simulink model "diff_controller"  (R2024b)
settings: Solver=FixedStepAuto  StartTime=0.0  StopTime=inf  FixedStep=0.001  RelTol=1e-3  EnableMultiTasking=on
InitFcn:
  | Ts = 0.005;
  | diameter = 165; %mm
  | width = 441; %mm
libraries: arduinolib x19, simulink x10, svdutilitieslib x5, simulink_extras x3, arduinosensorlib x2, robotmobilelib x1
(part 1 of 2)
settings Model: ExtModeTrigDuration=2  Creator=System-10  LastModifiedBy=01149
settings SolverCC: AutoInsertRateTranBlk=on
settings OptimizationCC: EnhancedBackFolding=on  PassReuseOutputArgsAs=Individual arguments  ZeroExternalMemoryAtStartup=off  ZeroInternalMemoryAtStartup=off  MaxStackSize=64  OptimizeBlockOrder=speed  DifferentSizesBufferReuse=on  OptimizationCustomize=off  EfficientTunableParamExpr=on
settings DebuggingCC: ParameterTunabilityLossMsg=error
settings HardwareCC: ProdBitPerInt=16  ProdBitPerPointer=16  ProdBitPerSizeT=16  ProdBitPerPtrDiffT=16  ProdLargestAtomicFloat=None  ProdWordSize=8  ProdHWDeviceType=Atmel->AVR
settings SFSimCC: MATLABDynamicMemAlloc=off
settings RTWCC: Description=Embedded Coder  SystemTargetFile=ert.tlc  HardwareBoard=Arduino Mega 2560  TemplateMakefile=ert_default_tmf  GenerateReport=on  Toolchain=Arduino AVR  BuildConfiguration=Faster Runs  GPUComputeCapability=3.5
settings CodeAppCC: ForceParamTrailComments=on  IgnoreCustomStorageClasses=off  OperatorAnnotations=on  SimulinkDataObjDesc=on  SFDataObjDesc=on  InsertBlockDesc=on
settings ERTTargetCC: SupportContinuousTime=on  SupportVariableSizeSignals=on  ExtModeTransport=3  ExtModeStaticAlloc=on  ExtModeAutomaticAllocSize=off  ExtModeStaticAllocSize=2048  ExtModeMexFile=ext_xcp  ExtModeIntrfLevel=Level2 - Open  InlinedParameterPlacement=Hierarchical  DynamicArrayContainerType=coder::array

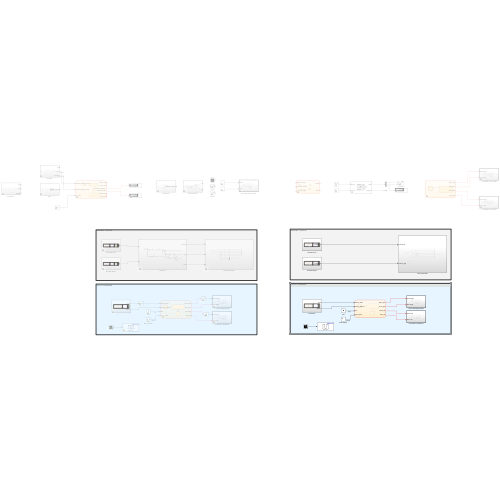
[thumbnail: Simulink's stored preview of the top-level diagram]
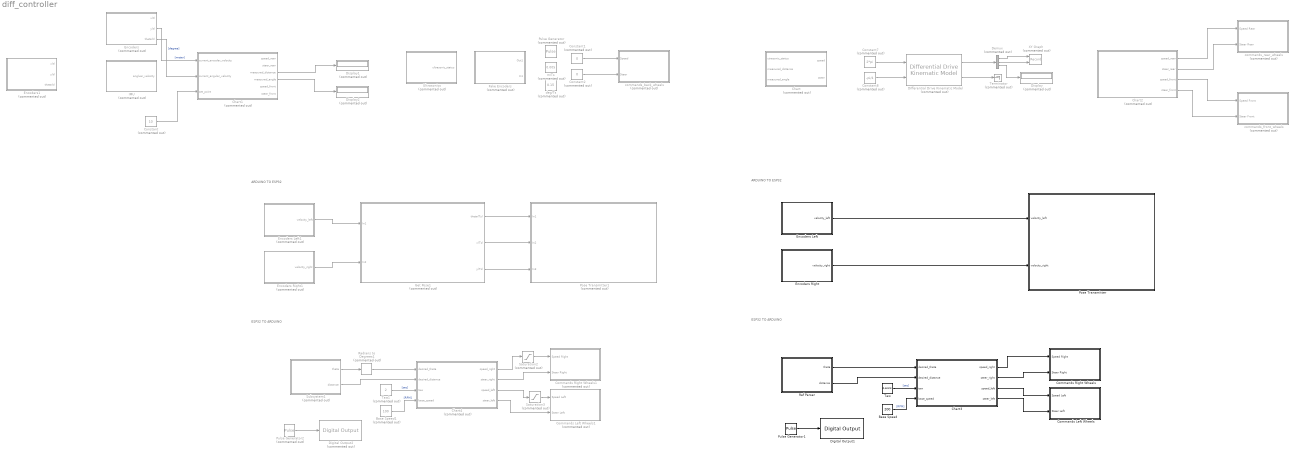
== system diff_controller ==
  note: ARDUINO TO ESP32
  note: ESP32 TO ARDUINO
  note: ESP32 TO ARDUINO
  note: ARDUINO TO ESP32
  Base Speed : Constant  Value=200  SampleTime=Ts
  Base Speed1 : Constant  Commented=on  Value=100  SampleTime=Ts
  Chart : Stateflow chart  Commented=on  TreatAsAtomicUnit=on
  Chart1 : Stateflow chart  Commented=on  TreatAsAtomicUnit=on
      settings: PortSchema="{\"entries\":[{\"content\":{\"sides\":[{\"content\":{\"connectorIds\":[\"In1\",\"In2\",\"In3\"]},\"type\":\"ConnectorPlacement.EquallySpacedRectSide\",\"uuid\":\"a18cf0c3-3c77-458c-bb3e-450a9e5c4723\"},{\"content\":{\"connectorIds\":[\"Out1\",\"Out2\",\"Out3\",\"Out6\",\"Out4\",\"Out5\"],\"side\":\"RIGHT\"},\"type\":\"ConnectorPlacement.EquallySpacedRectSide\",\"uuid\":\"c8115a23-9c0e-4673-86fd-819843dfe009\"},{\"content\":{\"side\":\"TOP\"},\"type\":\"ConnectorPlacement.EquallySpacedRectSide\",\"uuid\":\"db8a9c60-5937-48dc-b510-5b8795ac680a\"}]},\"type\":\"ConnectorPlacement.EquallySpacedConnector\",\"uuid\":\"4f3d77b9-4394-4090-867a-c6b2685c3613\"}],\"packageUris\":[\"http://schema.mathworks.com/mf0/Connector/R2020b\"],\"version\":\"1.0\"}"
  Chart2 : Stateflow chart  Commented=on  TreatAsAtomicUnit=on
  Chart3 : Stateflow chart  TreatAsAtomicUnit=on
  Chart4 : Stateflow chart  Commented=on  TreatAsAtomicUnit=on
  Commands Left Wheels : Subsystem  TreatAsAtomicUnit=on  SystemSampleTime=Ts
  Commands Left Wheels1 : Subsystem  Commented=on  TreatAsAtomicUnit=on  SystemSampleTime=0.1
  Commands Right Wheels : Subsystem  TreatAsAtomicUnit=on  SystemSampleTime=Ts
  Commands Right Wheels1 : Subsystem  Commented=on  TreatAsAtomicUnit=on  SystemSampleTime=0.1
  Constant : Constant  Commented=on  Value=10  SampleTime=Ts
  Constant1 : Constant  Commented=on  Value=0
  Constant2 : Constant  Commented=on  Value=0
  Constant7 : Constant  Commented=on  Value=2*pi
  Constant8 : Constant  Commented=on  Value=-pi/4
  Demux : Demux  Commented=on  Outputs=3
  Differential Drive Kinematic Model : robotmobilelib/Differential Drive Kinematic Model  Commented=on  VehicleInputs=Wheel Speeds  WheelRadius=0.165/2  WheelSpeedRange=[-inf inf]  TrackWidth=0.3  InitialState=[0; 0; 0]  SimulateUsing=Interpreted execution
  Digital Output1 : arduinolib/Digital Output  pinNumber=13  Direction=output  blockPlatform=arduino
  Digital Output2 : arduinolib/Digital Output  Commented=on  pinNumber=13  Direction=output  blockPlatform=arduino
  Display : Display  Commented=on
  Display1 : Display  Commented=on
  Display2 : Display  Commented=on
  Encoders : Subsystem  Commented=on
  Encoders Left : Subsystem
  Encoders Left1 : Subsystem  Commented=on
  Encoders Right : Subsystem
  Encoders Right1 : Subsystem  Commented=on
  Encoders1 : Subsystem  Commented=on
  Fake Encoders : Subsystem  Commented=on
      settings: PortSchema="{\"entries\":[{\"content\":{\"sides\":[{\"content\":{\"connectorIds\":[]},\"type\":\"ConnectorPlacement.EquallySpacedRectSide\",\"uuid\":\"5cdba24b-5905-4a96-853c-bd863ba68c1d\"},{\"content\":{\"connectorIds\":[\"Out1\",\"In1\"],\"side\":\"RIGHT\"},\"type\":\"ConnectorPlacement.EquallySpacedRectSide\",\"uuid\":\"1b3e1760-7d24-420c-94f1-a4f3cc053a4a\"},{\"content\":{\"connectorIds\":[],\"side\":\"TOP\"},\"type\":\"ConnectorPlacement.EquallySpacedRectSide\",\"uuid\":\"7746f2cc-443e-49dd-8fef-a3e999a80c85\"}]},\"type\":\"ConnectorPlacement.EquallySpacedConnector\",\"uuid\":\"959d968a-ce2e-4fe1-8e27-461b22c2fd96\"}],\"packageUris\":[\"http://schema.mathworks.com/mf0/Connector/R2020b\"],\"version\":\"1.0\"}"
  Get Pose1 : Subsystem  Commented=on
  IMU : Subsystem  Commented=on
  Pose Transmitter : Subsystem
  Pose Transmitter1 : Subsystem  Commented=on
  Pulse Generator : DiscretePulseGenerator  Commented=on  PulseType=Time based  Period=10  PulseWidth=20  PhaseDelay=10
  Pulse Generator1 : DiscretePulseGenerator  PulseType=Time based  PulseWidth=50
  Pulse Generator2 : DiscretePulseGenerator  Commented=on  PulseType=Time based  PulseWidth=50
  Radians to Degrees1 : simulink_extras/Transformations/Radians to Degrees  Commented=on
  Ref Parser : Subsystem
  Saturation2 : Saturate  Commented=on  UpperLimit=200  LowerLimit=-200
  Saturation3 : Saturate  Commented=on  UpperLimit=200  LowerLimit=-200
  Subsystem1 : Subsystem  Commented=on
  Taw : Constant  Value=0.441*3  SampleTime=Ts
  Taw1 : Constant  Commented=on  Value=2  SampleTime=Ts
  Terminator : Terminator  Commented=on
  Ultrasonics : Subsystem  Commented=on
  XY Graph : Record  Commented=on  FileSettingsInternal="{\"entries\":[{\"content\":{\"excelSettings\":{\"content\":{},\"type\":\"Streamout.ExcelSettings\"}},\"type\":\"Streamout.FileSettingStorage\",\"uuid\":\"\"}],\"packageUris\":[\"http:\\/\\/schema.mathworks.com\\/mf0\\/streamout_blocks\\/R2020a\"],\"version\":\"1.0\"}"  Layout=[1 1]  SignalsInternal="{\"entries\":[{\"content\":{\"signals\":[{\"content\":{\"blockPath\":[],\"dimensions\":[1],\"domain\":\"\",\"lineColor\":\"#a2142f\",\"plots\":[ 1 ],\"port\":1,\"signalID\":1,\"signalName\":\"Demux:1\"},\"type\":\"RecordBlkView.Signal\",\"uuid\":\"\"},{\"content\":{\"blockPath\":[],\"dimensions\":[1],\"domain\":\"\",\"lineColor\":\"#139fff\",\"plots\":[ 1 ],\"port\":2,\"signalID\":2,\"signalName\":\"Demux:2\"},\"type\":\"RecordBlkView.Signal\",\"uuid\":\"\"}]},\"type\":\"RecordBlkView.InputSignals\",\"uuid\":\"\"}],\"packageUris\":[\"http:\\/\\/schema.mathworks.com\\/mf0\\/streamout_blocks\\/R2020a\"],\"version\":\"1.0\"}"  VisualizationBindings="{\"xyplotplugin\":{\"info\":[{\"series\":[{\"bindingParametersList\":[{\"parameter\":\"X-Axis\",\"signalID\":1,\"signalName\":\"Demux:1\"},{\"parameter\":\"Y-Axis\",\"signalID\":2,\"signalName\":\"Demux:2\"}],\"seriesID\":0}],\"subplotID\":1}]}}"  CompatibilityTag=XY
  commands_back_wheels : Subsystem  Commented=on  TreatAsAtomicUnit=on  SystemSampleTime=0.1
  commands_front_wheels : Subsystem  Commented=on  TreatAsAtomicUnit=on  SystemSampleTime=0.1
  commands_rear_wheels : Subsystem  Commented=on  TreatAsAtomicUnit=on  SystemSampleTime=0.1
  deg/Ts : Constant  Commented=on  Value=0.15
  m/Ts : Constant  Commented=on  Value=0.005
  wires:
  Constant/1 -> Chart1/3(set_point)
  Constant1/1 -> commands_back_wheels/1(Speed)
  Constant2/1 -> commands_back_wheels/2(Steer)
  Chart1/3(measured_distance) -> Display1/1
  Chart1/6(measured_angle) -> Display2/1
  Differential Drive Kinematic Model/2 -> Terminator/1
  Differential Drive Kinematic Model/1 -> Demux/1
  Constant7/1 -> Differential Drive Kinematic Model/1
  Constant8/1 -> Differential Drive Kinematic Model/2
  Demux/1 -> XY Graph/1
  Demux/2 -> XY Graph/2
  Demux/3 -> Display/1
  Encoders/2(y(t)) -> Chart1/1(current_encoder_velocity)  "[meter]"
  Encoders/3(theta(t)) -> Chart1/2(current_angular_velocity)  "[degree]"
  Chart2/1(speed_rear) -> commands_rear_wheels/1(Speed Rear)
  Chart2/2(steer_rear) -> commands_rear_wheels/2(Steer Rear)
  Chart2/3(speed_front) -> commands_front_wheels/1(Speed Front)
  Chart2/4(stear_front) -> commands_front_wheels/2(Steer Front)
  Pulse Generator2/1 -> Digital Output2/1
  Encoders Left1/1(velocity_left) -> Get Pose1/1(In1)
  Chart4/4(steer_left) -> Commands Left Wheels1/2(Steer Left)
  Subsystem1/1(theta) -> Radians to Degrees1/1
  Get Pose1/1(theta(Ts)) -> Pose Transmitter1/1(In1)
  Get Pose1/2(x(Ts)) -> Pose Transmitter1/2(In2)
  Base Speed1/1 -> Chart4/4(base_speed)  "[RPM]"
  Chart4/2(steer_right) -> Commands Right Wheels1/2(Steer Right)
  Chart4/1(speed_right) -> Saturation2/1
  Encoders Right1/1(velocity_right) -> Get Pose1/2(In2)
  Saturation3/1 -> Commands Left Wheels1/1(Speed Left)
  Taw1/1 -> Chart4/3(taw)  "[sec]"
  Saturation2/1 -> Commands Right Wheels1/1(Speed Right)
  Chart4/3(speed_left) -> Saturation3/1
  Get Pose1/3(y(Ts)) -> Pose Transmitter1/3(In3)
  Subsystem1/2(distance) -> Chart4/2(desired_distance)
  Radians to Degrees1/1 -> Chart4/1(desired_theta)
  Chart3/1(speed_right) -> Commands Right Wheels/1(Speed Right)
  Chart3/3(speed_left) -> Commands Left Wheels/1(Speed Left)
  Chart3/2(steer_right) -> Commands Right Wheels/2(Steer Right)
  Chart3/4(steer_left) -> Commands Left Wheels/2(Steer Left)
  Base Speed/1 -> Chart3/4(base_speed)  "[RPM]"
  Pulse Generator1/1 -> Digital Output1/1
  Taw/1 -> Chart3/3(taw)  "[sec]"
  Encoders Left/1(velocity_left) -> Pose Transmitter/1(velocity_left)
  Encoders Right/1(velocity_right) -> Pose Transmitter/2(velocity_right)
  Ref Parser/1(theta) -> Chart3/1(desired_theta)
  Ref Parser/2(distance) -> Chart3/2(desired_distance)

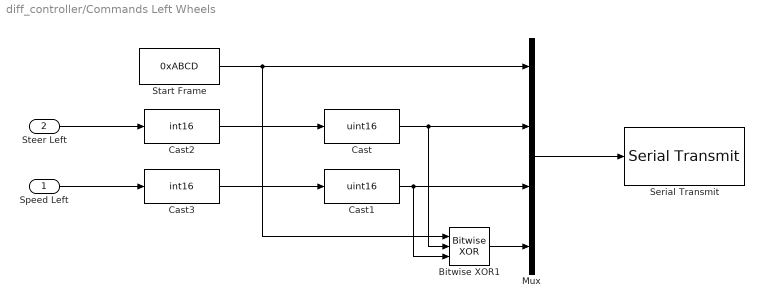
== system diff_controller/Commands Left Wheels ==
  Speed Left : Inport
  Steer Left : Inport  Port=2
  Bitwise XOR1 : simulink/Logic and Bit Operations/Bitwise Operator  logicop=XOR  UseBitMask=off  NumInputPorts=3  BitMask=bin2dec('11011001')  BitMaskRealWorld=Stored Integer
      settings: LibrarySourceBlock=|
      | simulink/Quick Insert/Logic and Bit
      | Operations/Bitwise XOR
  Cast : DataTypeConversion  OutDataTypeStr=uint16  SaturateOnIntegerOverflow=off  RndMeth=Floor
  Cast1 : DataTypeConversion  OutDataTypeStr=uint16  SaturateOnIntegerOverflow=off  RndMeth=Floor
  Cast2 : DataTypeConversion  OutDataTypeStr=int16  SaturateOnIntegerOverflow=off  RndMeth=Floor
  Cast3 : DataTypeConversion  OutDataTypeStr=int16  SaturateOnIntegerOverflow=off  RndMeth=Floor
  Mux : Mux
  Serial Transmit : arduinolib/Serial Transmit  portNumber=3  sendmode=write  sendformat=Decimal  floatprecision=2  header=[]  terminator=[]  blockPlatform=arduino
  Start Frame : Constant  Value=0xABCD  OutDataTypeStr=uint16
  wires:
  Cast1/1 -> Bitwise XOR1/3, Mux/3
  Speed Left/1 -> Cast3/1
  Start Frame/1 -> Bitwise XOR1/1, Mux/1
  Mux/1 -> Serial Transmit/1
  Steer Left/1 -> Cast2/1
  Bitwise XOR1/1 -> Mux/4
  Cast/1 -> Bitwise XOR1/2, Mux/2
  Cast2/1 -> Cast/1
  Cast3/1 -> Cast1/1

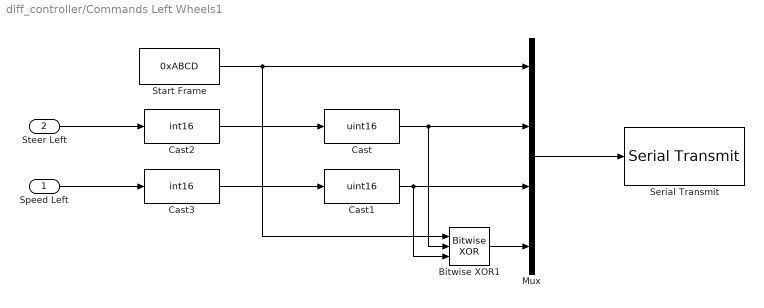
== system diff_controller/Commands Left Wheels1 ==
  Speed Left : Inport
  Steer Left : Inport  Port=2
  Bitwise XOR1 : simulink/Logic and Bit Operations/Bitwise Operator  logicop=XOR  UseBitMask=off  NumInputPorts=3  BitMask=bin2dec('11011001')  BitMaskRealWorld=Stored Integer
      settings: LibrarySourceBlock=|
      | simulink/Quick Insert/Logic and Bit
      | Operations/Bitwise XOR
  Cast : DataTypeConversion  OutDataTypeStr=uint16  SaturateOnIntegerOverflow=off  RndMeth=Floor
  Cast1 : DataTypeConversion  OutDataTypeStr=uint16  SaturateOnIntegerOverflow=off  RndMeth=Floor
  Cast2 : DataTypeConversion  OutDataTypeStr=int16  SaturateOnIntegerOverflow=off  RndMeth=Floor
  Cast3 : DataTypeConversion  OutDataTypeStr=int16  SaturateOnIntegerOverflow=off  RndMeth=Floor
  Mux : Mux
  Serial Transmit : arduinolib/Serial Transmit  portNumber=3  sendmode=write  sendformat=Decimal  floatprecision=2  header=[]  terminator=[]  blockPlatform=arduino
  Start Frame : Constant  Value=0xABCD  OutDataTypeStr=uint16
  wires:
  Cast1/1 -> Bitwise XOR1/3, Mux/3
  Speed Left/1 -> Cast3/1
  Start Frame/1 -> Bitwise XOR1/1, Mux/1
  Mux/1 -> Serial Transmit/1
  Steer Left/1 -> Cast2/1
  Bitwise XOR1/1 -> Mux/4
  Cast/1 -> Bitwise XOR1/2, Mux/2
  Cast2/1 -> Cast/1
  Cast3/1 -> Cast1/1

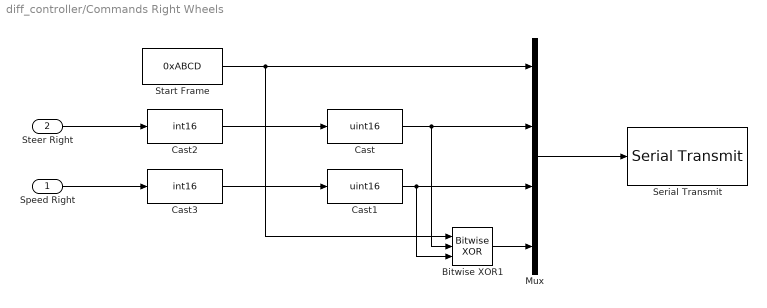
== system diff_controller/Commands Right Wheels ==
  Speed Right : Inport
  Steer Right : Inport  Port=2
  Bitwise XOR1 : simulink/Logic and Bit Operations/Bitwise Operator  logicop=XOR  UseBitMask=off  NumInputPorts=3  BitMask=bin2dec('11011001')  BitMaskRealWorld=Stored Integer
      settings: LibrarySourceBlock=|
      | simulink/Quick Insert/Logic and Bit
      | Operations/Bitwise XOR
  Cast : DataTypeConversion  OutDataTypeStr=uint16  SaturateOnIntegerOverflow=off  RndMeth=Floor
  Cast1 : DataTypeConversion  OutDataTypeStr=uint16  SaturateOnIntegerOverflow=off  RndMeth=Floor
  Cast2 : DataTypeConversion  OutDataTypeStr=int16  SaturateOnIntegerOverflow=off  RndMeth=Floor
  Cast3 : DataTypeConversion  OutDataTypeStr=int16  SaturateOnIntegerOverflow=off  RndMeth=Floor
  Mux : Mux
  Serial Transmit : arduinolib/Serial Transmit  portNumber=2  sendmode=write  sendformat=Decimal  floatprecision=2  header=[]  terminator=[]  blockPlatform=arduino
  Start Frame : Constant  Value=0xABCD  OutDataTypeStr=uint16
  wires:
  Cast1/1 -> Bitwise XOR1/3, Mux/3
  Speed Right/1 -> Cast3/1
  Start Frame/1 -> Bitwise XOR1/1, Mux/1
  Mux/1 -> Serial Transmit/1
  Steer Right/1 -> Cast2/1
  Bitwise XOR1/1 -> Mux/4
  Cast/1 -> Bitwise XOR1/2, Mux/2
  Cast2/1 -> Cast/1
  Cast3/1 -> Cast1/1

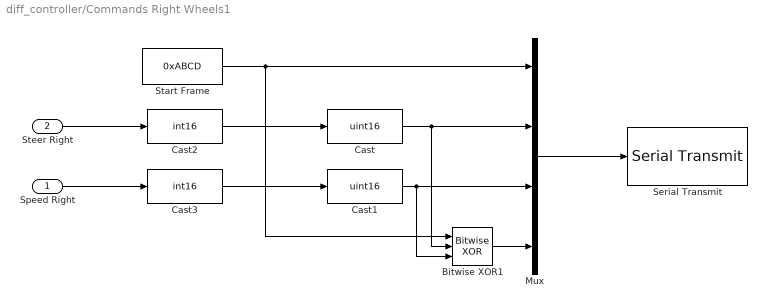
== system diff_controller/Commands Right Wheels1 ==
  Speed Right : Inport
  Steer Right : Inport  Port=2
  Bitwise XOR1 : simulink/Logic and Bit Operations/Bitwise Operator  logicop=XOR  UseBitMask=off  NumInputPorts=3  BitMask=bin2dec('11011001')  BitMaskRealWorld=Stored Integer
      settings: LibrarySourceBlock=|
      | simulink/Quick Insert/Logic and Bit
      | Operations/Bitwise XOR
  Cast : DataTypeConversion  OutDataTypeStr=uint16  SaturateOnIntegerOverflow=off  RndMeth=Floor
  Cast1 : DataTypeConversion  OutDataTypeStr=uint16  SaturateOnIntegerOverflow=off  RndMeth=Floor
  Cast2 : DataTypeConversion  OutDataTypeStr=int16  SaturateOnIntegerOverflow=off  RndMeth=Floor
  Cast3 : DataTypeConversion  OutDataTypeStr=int16  SaturateOnIntegerOverflow=off  RndMeth=Floor
  Mux : Mux
  Serial Transmit : arduinolib/Serial Transmit  portNumber=2  sendmode=write  sendformat=Decimal  floatprecision=2  header=[]  terminator=[]  blockPlatform=arduino
  Start Frame : Constant  Value=0xABCD  OutDataTypeStr=uint16
  wires:
  Cast1/1 -> Bitwise XOR1/3, Mux/3
  Speed Right/1 -> Cast3/1
  Start Frame/1 -> Bitwise XOR1/1, Mux/1
  Mux/1 -> Serial Transmit/1
  Steer Right/1 -> Cast2/1
  Bitwise XOR1/1 -> Mux/4
  Cast/1 -> Bitwise XOR1/2, Mux/2
  Cast2/1 -> Cast/1
  Cast3/1 -> Cast1/1

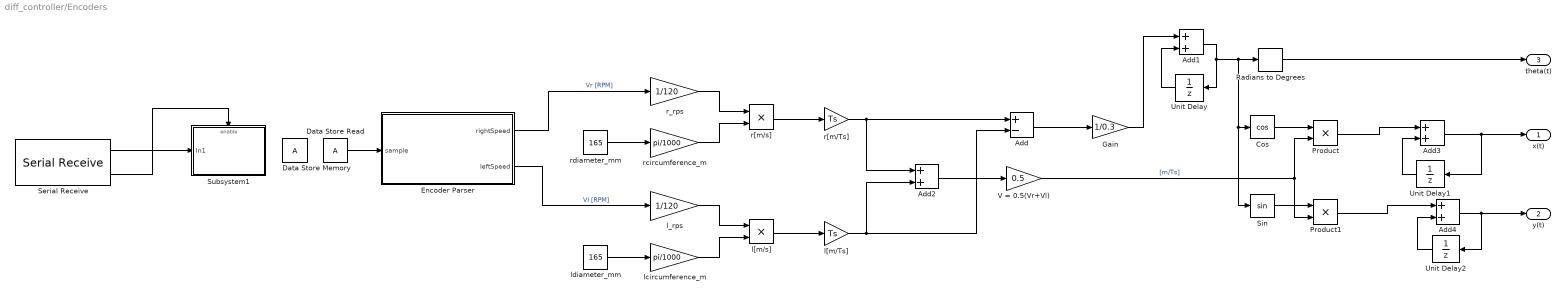
== system diff_controller/Encoders ==
  Add : Sum  Inputs=+-
  Add{1..4} (4 alike) : Sum
  Cos : Trigonometry  Operator=cos
  Data Store Memory : DataStoreMemory  WriteAfterWriteMsg=warning  InitialValue=88  ShowAdditionalParam=off  OutDataTypeStr=int16  Dimensions=[1 16]
  Data Store Read : DataStoreRead  IndexOptions=Index vector (dialog)  Indices=1  OutputSizes=1
  Encoder Parser : MATLAB Function  TreatAsAtomicUnit=on
  Gain : Gain  Gain=1/0.3
  Product : Product
  Product1 : Product
  Radians to Degrees : simulink_extras/Transformations/Radians to Degrees
  Serial Receive : arduinolib/Serial Receive  portNumber=1  DataType=int16  blockPlatform=arduino  TimeOut=0  MaxDataLength=10  isARMArch=off  DataLengthOption=Length via dialog  Datalength=16  Header=[]  Terminator=[]  SampleTime=Ts  ShowOutStatus=on
  Sin : Trigonometry
  Subsystem1 : Subsystem
  Unit Delay : UnitDelay  SampleTime=-1  HasFrameUpgradeWarning=on
  Unit Delay1 : UnitDelay  SampleTime=-1  HasFrameUpgradeWarning=on
  Unit Delay2 : UnitDelay  SampleTime=-1  HasFrameUpgradeWarning=on
  V = 0.5(Vr+Vl) : Gain  Gain=0.5
  l[m/Ts] : Gain  Gain=Ts
  l[m/s] : Product
  l_rps : Gain  Gain=1/120
  lcircumference_m : Gain  Gain=pi/1000
  ldiameter_mm : Constant  Value=165  SampleTime=Ts
  r[m/Ts] : Gain  Gain=Ts
  r[m/s] : Product
  r_rps : Gain  Gain=1/120
  rcircumference_m : Gain  Gain=pi/1000
  rdiameter_mm : Constant  Value=165  SampleTime=Ts
  x(t) : Outport
  y(t) : Outport  Port=2
  theta(t) : Outport  Port=3
  wires:
  Serial Receive/1 -> Subsystem1/1(In1)
  Data Store Read/1 -> Encoder Parser/1(sample)
  ldiameter_mm/1 -> lcircumference_m/1
  l_rps/1 -> l[m/s]/1
  lcircumference_m/1 -> l[m/s]/2
  Serial Receive/2 -> Subsystem1/Enable
  l[m/s]/1 -> l[m/Ts]/1
  rcircumference_m/1 -> r[m/s]/2
  r[m/s]/1 -> r[m/Ts]/1
  r_rps/1 -> r[m/s]/1
  rdiameter_mm/1 -> rcircumference_m/1
  Encoder Parser/1(rightSpeed) -> r_rps/1  "Vr [RPM]"
  Encoder Parser/2(leftSpeed) -> l_rps/1  "Vl [RPM]"
  Add/1 -> Gain/1
  Gain/1 -> Add1/1
  Add1/1 -> Sin/1, Cos/1, Radians to Degrees/1, Unit Delay/1
  Unit Delay/1 -> Add1/2
  Radians to Degrees/1 -> theta(t)/1
  r[m/Ts]/1 -> Add/1, Add2/1
  l[m/Ts]/1 -> Add2/2, Add/2
  Add2/1 -> V = 0.5(Vr+Vl)/1
  Cos/1 -> Product/1
  V = 0.5(Vr+Vl)/1 -> Product1/2, Product/2  "[m/Ts]"
  Sin/1 -> Product1/1
  Unit Delay1/1 -> Add3/2
  Unit Delay2/1 -> Add4/2
  Product/1 -> Add3/1
  Add3/1 -> Unit Delay1/1, x(t)/1
  Add4/1 -> Unit Delay2/1, y(t)/1
  Product1/1 -> Add4/1

== system diff_controller/Encoders Left ==
  note: OUTPUT
  note: DATA PARSING
  note: DATA ACQUISITION
  Data Store Memory : DataStoreMemory  WriteAfterWriteMsg=warning  InitialValue=88  ShowAdditionalParam=off  OutDataTypeStr=int16  Dimensions=[1 18]
  Data Store Read : DataStoreRead  IndexOptions=Index vector (dialog)  Indices=1  OutputSizes=1
  Encoder Parser : MATLAB Function  TreatAsAtomicUnit=on
  Serial Receive : arduinolib/Serial Receive  portNumber=3  DataType=int16  blockPlatform=arduino  TimeOut=0  MaxDataLength=10  isARMArch=off  DataLengthOption=Length via dialog  Datalength=18  Header=[]  Terminator=[]  SampleTime=Ts  ShowOutStatus=on
  Subsystem1 : Subsystem
  To Workspace : ToWorkspace  VariableName=port3_data  SampleTime=-1
      settings: Save2DSignal=2-D array (concatenate along first dimension)
  velocity_left : Outport
  wires:
  Serial Receive/1 -> To Workspace/1, Subsystem1/1(In1)
  Data Store Read/1 -> Encoder Parser/1(data)
  Serial Receive/2 -> Subsystem1/Enable
  Encoder Parser/1(averageSpeed) -> velocity_left/1  "Vl [RPM]"

== system diff_controller/Encoders Left1 ==
  note: OUTPUT
  note: CONVERSION
      | RPM => rad/s
      | *2*pi/60
      | rad/s => m/s
      | *pi*d
      | m/s => m/Ts
      | *Ts
  note: DATA PARSING
  note: DATA ACQUISITION
  Convert to [m/Ts] : Gain  Gain=2*(pi^2)*diameter*Ts/60000
  Data Store Memory : DataStoreMemory  WriteAfterWriteMsg=warning  InitialValue=88  ShowAdditionalParam=off  OutDataTypeStr=int16  Dimensions=[1 18]
  Data Store Read : DataStoreRead  IndexOptions=Index vector (dialog)  Indices=1  OutputSizes=1
  Encoder Parser : MATLAB Function  TreatAsAtomicUnit=on
  Serial Receive : arduinolib/Serial Receive  portNumber=3  DataType=int16  blockPlatform=arduino  TimeOut=0  MaxDataLength=10  isARMArch=off  DataLengthOption=Length via dialog  Datalength=18  Header=[]  Terminator=[]  SampleTime=Ts  ShowOutStatus=on
  Subsystem1 : Subsystem
  velocity_left : Outport
  wires:
  Serial Receive/1 -> Subsystem1/1(In1)
  Data Store Read/1 -> Encoder Parser/1(data)
  Serial Receive/2 -> Subsystem1/Enable
  Encoder Parser/1(averageSpeed) -> Convert to [m/Ts]/1  "Vl [RPM]"
  Convert to [m/Ts]/1 -> velocity_left/1  "[m/Ts]"

== system diff_controller/Encoders Right ==
  note: OUTPUT
  note: DATA PARSING
  note: DATA ACQUISITION
  Data Store Memory : DataStoreMemory  WriteAfterWriteMsg=warning  InitialValue=88  ShowAdditionalParam=off  OutDataTypeStr=int16  Dimensions=[1 18]
  Data Store Read : DataStoreRead  IndexOptions=Index vector (dialog)  Indices=1  OutputSizes=1
  Encoder Parser : MATLAB Function  TreatAsAtomicUnit=on
  Serial Receive : arduinolib/Serial Receive  portNumber=2  DataType=int16  blockPlatform=arduino  TimeOut=0  MaxDataLength=10  isARMArch=off  DataLengthOption=Length via dialog  Datalength=18  Header=[]  Terminator=[]  SampleTime=Ts  ShowOutStatus=on
  Subsystem1 : Subsystem
  To Workspace : ToWorkspace  VariableName=port2_data  SampleTime=-1
      settings: Save2DSignal=2-D array (concatenate along first dimension)
  velocity_right : Outport
  wires:
  Serial Receive/1 -> To Workspace/1, Subsystem1/1(In1)
  Data Store Read/1 -> Encoder Parser/1(data)
  Serial Receive/2 -> Subsystem1/Enable
  Encoder Parser/1(averageSpeed) -> velocity_right/1  "Vr [RPM]"

== system diff_controller/Encoders Right1 ==
  note: OUTPUT
  note: CONVERSION
      | RPM => rad/s
      | *2*pi/60
      | rad/s => m/s
      | *pi*d
      | m/s => m/Ts
      | *Ts
  note: DATA PARSING
  note: DATA ACQUISITION
  Data Store Memory : DataStoreMemory  WriteAfterWriteMsg=warning  InitialValue=88  ShowAdditionalParam=off  OutDataTypeStr=int16  Dimensions=[1 18]
  Data Store Read : DataStoreRead  IndexOptions=Index vector (dialog)  Indices=1  OutputSizes=1
  Encoder Parser : MATLAB Function  TreatAsAtomicUnit=on
  Serial Receive : arduinolib/Serial Receive  portNumber=2  DataType=int16  blockPlatform=arduino  TimeOut=0  MaxDataLength=10  isARMArch=off  DataLengthOption=Length via dialog  Datalength=18  Header=[]  Terminator=[]  SampleTime=Ts  ShowOutStatus=on
  Subsystem1 : Subsystem
  convert to  [m/Ts] : Gain  Gain=2*(pi^2)*diameter*Ts/60000
  velocity_right : Outport
  wires:
  Serial Receive/1 -> Subsystem1/1(In1)
  Data Store Read/1 -> Encoder Parser/1(data)
  Serial Receive/2 -> Subsystem1/Enable
  Encoder Parser/1(averageSpeed) -> convert to  [m/Ts]/1  "Vr [RPM]"
  convert to  [m/Ts]/1 -> velocity_right/1  "[m/Ts]"

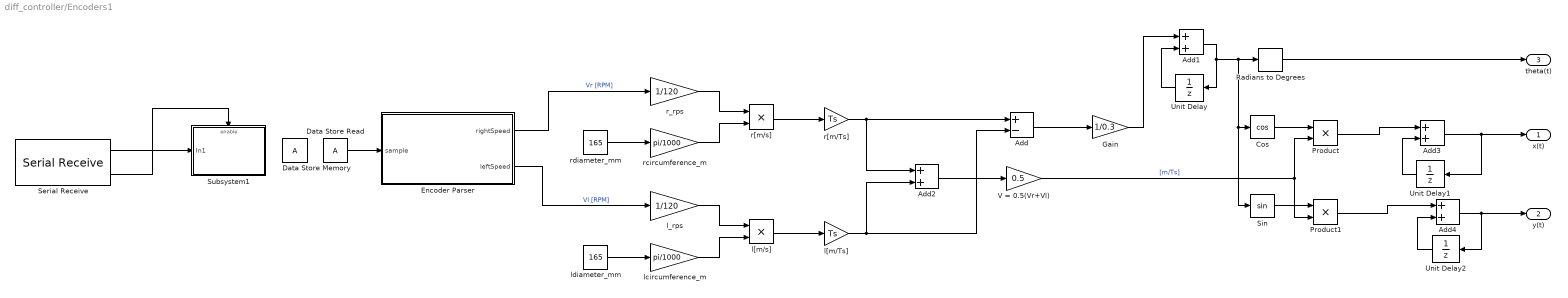
== system diff_controller/Encoders1 ==
  Add : Sum  Inputs=+-
  Add{1..4} (4 alike) : Sum
  Cos : Trigonometry  Operator=cos
  Data Store Memory : DataStoreMemory  WriteAfterWriteMsg=warning  InitialValue=88  ShowAdditionalParam=off  OutDataTypeStr=int16  Dimensions=[1 16]
  Data Store Read : DataStoreRead  IndexOptions=Index vector (dialog)  Indices=1  OutputSizes=1
  Encoder Parser : MATLAB Function  TreatAsAtomicUnit=on
  Gain : Gain  Gain=1/0.3
  Product : Product
  Product1 : Product
  Radians to Degrees : simulink_extras/Transformations/Radians to Degrees
  Serial Receive : arduinolib/Serial Receive  portNumber=1  DataType=int16  blockPlatform=arduino  TimeOut=0  MaxDataLength=10  isARMArch=off  DataLengthOption=Length via dialog  Datalength=16  Header=[]  Terminator=[]  SampleTime=Ts  ShowOutStatus=on
  Sin : Trigonometry
  Subsystem1 : Subsystem
  Unit Delay : UnitDelay  SampleTime=-1  HasFrameUpgradeWarning=on
  Unit Delay1 : UnitDelay  SampleTime=-1  HasFrameUpgradeWarning=on
  Unit Delay2 : UnitDelay  SampleTime=-1  HasFrameUpgradeWarning=on
  V = 0.5(Vr+Vl) : Gain  Gain=0.5
  l[m/Ts] : Gain  Gain=Ts
  l[m/s] : Product
  l_rps : Gain  Gain=1/120
  lcircumference_m : Gain  Gain=pi/1000
  ldiameter_mm : Constant  Value=165  SampleTime=Ts
  r[m/Ts] : Gain  Gain=Ts
  r[m/s] : Product
  r_rps : Gain  Gain=1/120
  rcircumference_m : Gain  Gain=pi/1000
  rdiameter_mm : Constant  Value=165  SampleTime=Ts
  x(t) : Outport
  y(t) : Outport  Port=2
  theta(t) : Outport  Port=3
  wires:
  Serial Receive/1 -> Subsystem1/1(In1)
  Data Store Read/1 -> Encoder Parser/1(sample)
  ldiameter_mm/1 -> lcircumference_m/1
  l_rps/1 -> l[m/s]/1
  lcircumference_m/1 -> l[m/s]/2
  Serial Receive/2 -> Subsystem1/Enable
  l[m/s]/1 -> l[m/Ts]/1
  rcircumference_m/1 -> r[m/s]/2
  r[m/s]/1 -> r[m/Ts]/1
  r_rps/1 -> r[m/s]/1
  rdiameter_mm/1 -> rcircumference_m/1
  Encoder Parser/1(rightSpeed) -> r_rps/1  "Vr [RPM]"
  Encoder Parser/2(leftSpeed) -> l_rps/1  "Vl [RPM]"
  Add/1 -> Gain/1
  Gain/1 -> Add1/1
  Add1/1 -> Sin/1, Cos/1, Radians to Degrees/1, Unit Delay/1
  Unit Delay/1 -> Add1/2
  Radians to Degrees/1 -> theta(t)/1
  r[m/Ts]/1 -> Add/1, Add2/1
  l[m/Ts]/1 -> Add2/2, Add/2
  Add2/1 -> V = 0.5(Vr+Vl)/1
  Cos/1 -> Product/1
  V = 0.5(Vr+Vl)/1 -> Product1/2, Product/2  "[m/Ts]"
  Sin/1 -> Product1/1
  Unit Delay1/1 -> Add3/2
  Unit Delay2/1 -> Add4/2
  Product/1 -> Add3/1
  Add3/1 -> Unit Delay1/1, x(t)/1
  Add4/1 -> Unit Delay2/1, y(t)/1
  Product1/1 -> Add4/1

== system diff_controller/Fake Encoders ==
  In1 : Inport
  Add : Sum
  Constant : Constant  Value=0
  Detect Increase : simulink/Logic and Bit Operations/Detect Increase  vinit=0.0  OutDataTypeStr=uint8
  Pulse Generator1 : DiscretePulseGenerator  PulseType=Time based  PulseWidth=5
  Switch : Switch  Criteria=u2 > Threshold  SaturateOnIntegerOverflow=off  InputSameDT=off
  Unit Delay : UnitDelay  SampleTime=-1  HasFrameUpgradeWarning=on
  Out1 : Outport
  wires:
  Add/1 -> Out1/1, Unit Delay/1
  Pulse Generator1/1 -> Detect Increase/1
  Constant/1 -> Switch/3
  Detect Increase/1 -> Switch/1
  Unit Delay/1 -> Add/2
  Switch/1 -> Add/1
  In1/1 -> Switch/2

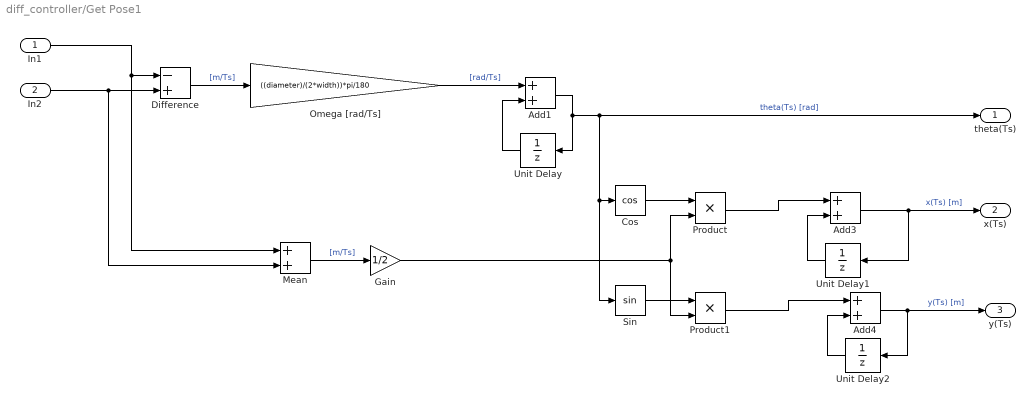
== system diff_controller/Get Pose1 ==
  In1 : Inport
  In2 : Inport  Port=2
  Add1 : Sum
  Add3 : Sum
  Add4 : Sum
  Cos : Trigonometry  Operator=cos
  Difference : Sum  Inputs=-+
  Gain : Gain  Gain=1/2
  Mean : Sum
  Omega [rad/Ts] : Gain  Gain=((diameter)/(2*width))*pi/180
  Product : Product
  Product1 : Product
  Sin : Trigonometry
  Unit Delay : UnitDelay  SampleTime=-1  HasFrameUpgradeWarning=on
  Unit Delay1 : UnitDelay  SampleTime=-1  HasFrameUpgradeWarning=on
  Unit Delay2 : UnitDelay  SampleTime=-1  HasFrameUpgradeWarning=on
  theta(Ts) : Outport
  x(Ts) : Outport  Port=2
  y(Ts) : Outport  Port=3
  wires:
  Add1/1 -> theta(Ts)/1, Sin/1, Cos/1, Unit Delay/1  "theta(Ts) [rad]"
  Add3/1 -> x(Ts)/1, Unit Delay1/1  "x(Ts) [m]"
  Omega [rad/Ts]/1 -> Add1/1  "[rad/Ts]"
  Unit Delay2/1 -> Add4/2
  Difference/1 -> Omega [rad/Ts]/1  "[m/Ts]"
  Add4/1 -> y(Ts)/1, Unit Delay2/1  "y(Ts) [m]"
  Gain/1 -> Product/2, Product1/2
  Product1/1 -> Add4/1
  Unit Delay/1 -> Add1/2
  Unit Delay1/1 -> Add3/2
  Cos/1 -> Product/1
  Product/1 -> Add3/1
  In1/1 -> Difference/1, Mean/1
  Sin/1 -> Product1/1
  In2/1 -> Mean/2, Difference/2
  Mean/1 -> Gain/1  "[m/Ts]"

== system diff_controller/IMU ==
  Demux : Demux  Outputs=3
  Gain : Gain  Gain=Ts
  MPU6050 IMU Sensor : arduinosensorlib/MPU6050 IMU Sensor  I2CModule=0  SlaveAddress=0x68  Accel=off  AngularRate=on  Temperature=off  Status=off  Timestamp=off  EulerAngles=off  Quat=off  AccelRange=2G  GyroRange=250 dps  DmpOdr=200 Hz  Dlpf=Accelerometer: 184Hz, Gyroscope: 188Hz  spf=1  SampleTime=-1  QueueSizeFactor=1
  Terminator : Terminator
  Terminator1 : Terminator
  angluar_velocity : Outport
  wires:
  MPU6050 IMU Sensor/1 -> Demux/1
  Demux/1 -> Terminator/1
  Demux/2 -> Terminator1/1
  Demux/3 -> Gain/1
  Gain/1 -> angluar_velocity/1

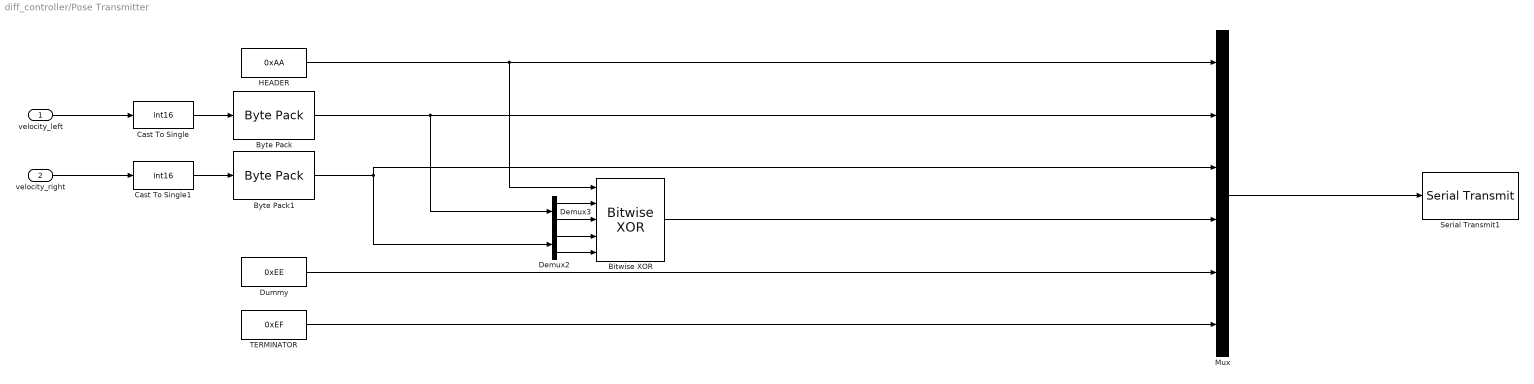
== system diff_controller/Pose Transmitter ==
  velocity_left : Inport
  velocity_right : Inport  Port=2
  Bitwise XOR : simulink/Logic and Bit Operations/Bitwise Operator  logicop=XOR  UseBitMask=off  NumInputPorts=5  BitMask=bin2dec('11011001')  BitMaskRealWorld=Stored Integer
      settings: LibrarySourceBlock=|
      | simulink/Quick Insert/Logic and Bit
      | Operations/Bitwise XOR
  Byte Pack : svdutilitieslib/Byte Pack  maskPackedDataType=uint8  datatypes={'int16'}  byteAlign=1  blockPlatform=arduinoert
  Byte Pack1 : svdutilitieslib/Byte Pack  maskPackedDataType=uint8  datatypes={'int16'}  byteAlign=1  blockPlatform=arduinoert
  Cast To Single : DataTypeConversion  OutDataTypeStr=int16  SaturateOnIntegerOverflow=off  RndMeth=Floor
  Cast To Single1 : DataTypeConversion  OutDataTypeStr=int16  SaturateOnIntegerOverflow=off  RndMeth=Floor
  Demux2 : Demux  Outputs=2
  Demux3 : Demux  Outputs=2
  Dummy : Constant  Value=0xEE  OutDataTypeStr=uint8  SampleTime=Ts
  HEADER : Constant  Value=0xAA  OutDataTypeStr=uint8  SampleTime=Ts
  Mux : Mux  Inputs=6
  Serial Transmit1 : arduinolib/Serial Transmit  portNumber=1  sendmode=write  sendformat=Decimal  floatprecision=2  header=[]  terminator=[]  blockPlatform=arduino
  TERMINATOR : Constant  Value=0xEF  OutDataTypeStr=uint8  SampleTime=Ts
  wires:
  velocity_right/1 -> Cast To Single1/1
  Mux/1 -> Serial Transmit1/1
  HEADER/1 -> Bitwise XOR/1, Mux/1
  Byte Pack/1 -> Demux3/1, Mux/2
  Byte Pack1/1 -> Demux2/1, Mux/3
  TERMINATOR/1 -> Mux/6
  Bitwise XOR/1 -> Mux/4
  Dummy/1 -> Mux/5
  velocity_left/1 -> Cast To Single/1
  Demux2/2 -> Bitwise XOR/5
  Demux2/1 -> Bitwise XOR/4
  Demux3/1 -> Bitwise XOR/2
  Demux3/2 -> Bitwise XOR/3
  Cast To Single1/1 -> Byte Pack1/1
  Cast To Single/1 -> Byte Pack/1

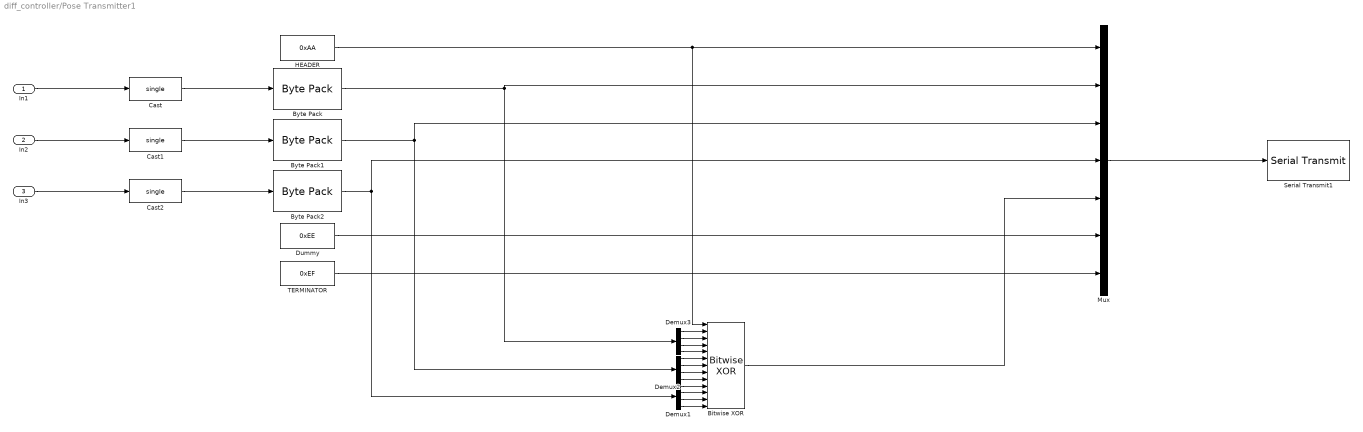
== system diff_controller/Pose Transmitter1 ==
  In1 : Inport
  In2 : Inport  Port=2
  In3 : Inport  Port=3
  Bitwise XOR : simulink/Logic and Bit Operations/Bitwise Operator  logicop=XOR  UseBitMask=off  NumInputPorts=13  BitMask=bin2dec('11011001')  BitMaskRealWorld=Stored Integer
      settings: LibrarySourceBlock=|
      | simulink/Quick Insert/Logic and Bit
      | Operations/Bitwise XOR
  Byte Pack : svdutilitieslib/Byte Pack  maskPackedDataType=uint8  datatypes={'single'}  byteAlign=1  blockPlatform=arduinoert
  Byte Pack1 : svdutilitieslib/Byte Pack  maskPackedDataType=uint8  datatypes={'single'}  byteAlign=1  blockPlatform=arduinoert
  Byte Pack2 : svdutilitieslib/Byte Pack  maskPackedDataType=uint8  datatypes={'single'}  byteAlign=1  blockPlatform=arduinoert
  Cast : DataTypeConversion  OutDataTypeStr=single  SaturateOnIntegerOverflow=off  RndMeth=Floor
  Cast1 : DataTypeConversion  OutDataTypeStr=single  SaturateOnIntegerOverflow=off  RndMeth=Floor
  Cast2 : DataTypeConversion  OutDataTypeStr=single  SaturateOnIntegerOverflow=off  RndMeth=Floor
  Demux1 : Demux
  Demux2 : Demux
  Demux3 : Demux
  Dummy : Constant  Value=0xEE  OutDataTypeStr=uint8  SampleTime=Ts
  HEADER : Constant  Value=0xAA  OutDataTypeStr=uint8  SampleTime=Ts
  Mux : Mux  Inputs=7
  Serial Transmit1 : arduinolib/Serial Transmit  portNumber=1  sendmode=write  sendformat=Decimal  floatprecision=2  header=[]  terminator=[]  blockPlatform=arduino
  TERMINATOR : Constant  Value=0xEF  OutDataTypeStr=uint8  SampleTime=Ts
  wires:
  Cast1/1 -> Byte Pack1/1
  Demux3/3 -> Bitwise XOR/4
  Demux3/1 -> Bitwise XOR/2
  Cast2/1 -> Byte Pack2/1
  Bitwise XOR/1 -> Mux/5
  Byte Pack2/1 -> Mux/4, Demux1/1
  HEADER/1 -> Bitwise XOR/1, Mux/1
  Demux1/3 -> Bitwise XOR/12
  Demux1/4 -> Bitwise XOR/13
  Cast/1 -> Byte Pack/1
  Mux/1 -> Serial Transmit1/1
  In3/1 -> Cast2/1
  Dummy/1 -> Mux/6
  Demux2/3 -> Bitwise XOR/8
  Demux3/2 -> Bitwise XOR/3
  Byte Pack/1 -> Demux3/1, Mux/2
  TERMINATOR/1 -> Mux/7
  Demux1/1 -> Bitwise XOR/10
  Demux1/2 -> Bitwise XOR/11
  Demux2/2 -> Bitwise XOR/7
  Demux3/4 -> Bitwise XOR/5
  Demux2/4 -> Bitwise XOR/9
  Demux2/1 -> Bitwise XOR/6
  Byte Pack1/1 -> Mux/3, Demux2/1
  In2/1 -> Cast1/1
  In1/1 -> Cast/1

== system diff_controller/Ref Parser ==
  note: DATA ACQUISITION
  note: DATA PARSING
  note: OUTPUT
  Data Store Memory : DataStoreMemory  WriteAfterWriteMsg=warning  InitialValue=88  ShowAdditionalParam=off  OutDataTypeStr=uint8  Dimensions=[1 24]
  Data Store Read : DataStoreRead  IndexOptions=Index vector (dialog)  Indices=1  OutputSizes=1
  Ref Parser : MATLAB Function  TreatAsAtomicUnit=on
  Serial Receive : arduinolib/Serial Receive  portNumber=1  DataType=uint8  blockPlatform=arduino  TimeOut=10  MaxDataLength=16  isARMArch=off  DataLengthOption=Length via dialog  Datalength=24  Header=[]  Terminator=[]  SampleTime=Ts  ShowOutStatus=on
  Subsystem1 : Subsystem
  theta : Outport
  distance : Outport  Port=2
  wires:
  Serial Receive/2 -> Subsystem1/Enable
  Data Store Read/1 -> Ref Parser/1(data)
  Serial Receive/1 -> Subsystem1/1(In1)
  Ref Parser/1(theta) -> theta/1
  Ref Parser/2(distance) -> distance/1

== system diff_controller/Subsystem1 ==
  note: DATA ACQUISITION
  note: DATA PARSING
  note: OUTPUT
  Data Store Memory : DataStoreMemory  WriteAfterWriteMsg=warning  InitialValue=88  ShowAdditionalParam=off  OutDataTypeStr=uint8  Dimensions=[1 24]
  Data Store Read : DataStoreRead  IndexOptions=Index vector (dialog)  Indices=1  OutputSizes=1
  Pose Parser : MATLAB Function  TreatAsAtomicUnit=on
  Serial Receive : arduinolib/Serial Receive  portNumber=1  DataType=uint8  blockPlatform=arduino  TimeOut=10  MaxDataLength=16  isARMArch=off  DataLengthOption=Length via dialog  Datalength=24  Header=[]  Terminator=[]  SampleTime=Ts  ShowOutStatus=on
  Subsystem1 : Subsystem
  theta : Outport
  distance : Outport  Port=2
  wires:
  Serial Receive/2 -> Subsystem1/Enable
  Data Store Read/1 -> Pose Parser/1(data)
  Serial Receive/1 -> Subsystem1/1(In1)
  Pose Parser/1(theta) -> theta/1
  Pose Parser/2(distance) -> distance/1

== system diff_controller/Ultrasonics ==
  Constant : Constant  Value=0  OutDataTypeStr=boolean
  Constant1 : Constant  OutDataTypeStr=boolean
  Switch : Switch  Criteria=u2 > Threshold  Threshold=2  SaturateOnIntegerOverflow=off  InputSameDT=off
  Ultrasonic Sensor : arduinosensorlib/Ultrasonic Sensor  NumSignalPins=2  TrigPin=4  EchoPin=5  SignalPin=3  SampleTime_=Ts  blockPlatform=ARDUINO
  ultrasonic_status : Outport
  wires:
  Ultrasonic Sensor/1 -> Switch/2
  Constant/1 -> Switch/1
  Constant1/1 -> Switch/3
  Switch/1 -> ultrasonic_status/1

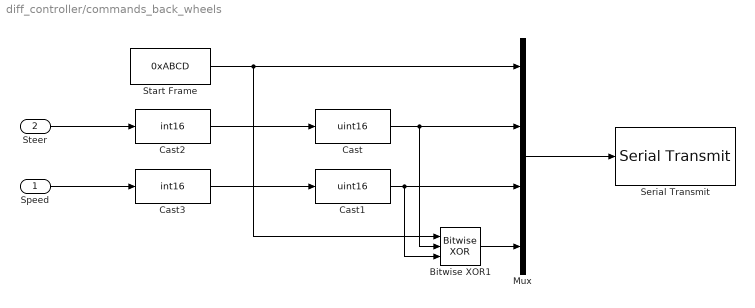
== system diff_controller/commands_back_wheels ==
  Speed : Inport
  Steer : Inport  Port=2
  Bitwise XOR1 : simulink/Logic and Bit Operations/Bitwise Operator  logicop=XOR  UseBitMask=off  NumInputPorts=3  BitMask=bin2dec('11011001')  BitMaskRealWorld=Stored Integer
      settings: LibrarySourceBlock=|
      | simulink/Quick Insert/Logic and Bit
      | Operations/Bitwise XOR
  Cast : DataTypeConversion  OutDataTypeStr=uint16  SaturateOnIntegerOverflow=off  RndMeth=Floor
  Cast1 : DataTypeConversion  OutDataTypeStr=uint16  SaturateOnIntegerOverflow=off  RndMeth=Floor
  Cast2 : DataTypeConversion  OutDataTypeStr=int16  SaturateOnIntegerOverflow=off  RndMeth=Floor
  Cast3 : DataTypeConversion  OutDataTypeStr=int16  SaturateOnIntegerOverflow=off  RndMeth=Floor
  Mux : Mux
  Serial Transmit : arduinolib/Serial Transmit  portNumber=1  sendmode=write  sendformat=Decimal  floatprecision=2  blockPlatform=arduino
  Start Frame : Constant  Value=0xABCD  OutDataTypeStr=uint16
  wires:
  Cast1/1 -> Bitwise XOR1/3, Mux/3
  Speed/1 -> Cast3/1
  Start Frame/1 -> Bitwise XOR1/1, Mux/1
  Mux/1 -> Serial Transmit/1
  Steer/1 -> Cast2/1
  Bitwise XOR1/1 -> Mux/4
  Cast/1 -> Bitwise XOR1/2, Mux/2
  Cast2/1 -> Cast/1
  Cast3/1 -> Cast1/1

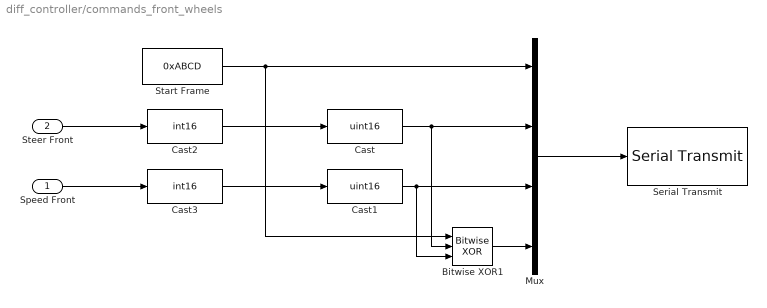
== system diff_controller/commands_front_wheels ==
  Speed Front : Inport
  Steer Front : Inport  Port=2
  Bitwise XOR1 : simulink/Logic and Bit Operations/Bitwise Operator  logicop=XOR  UseBitMask=off  NumInputPorts=3  BitMask=bin2dec('11011001')  BitMaskRealWorld=Stored Integer
      settings: LibrarySourceBlock=|
      | simulink/Quick Insert/Logic and Bit
      | Operations/Bitwise XOR
  Cast : DataTypeConversion  OutDataTypeStr=uint16  SaturateOnIntegerOverflow=off  RndMeth=Floor
  Cast1 : DataTypeConversion  OutDataTypeStr=uint16  SaturateOnIntegerOverflow=off  RndMeth=Floor
  Cast2 : DataTypeConversion  OutDataTypeStr=int16  SaturateOnIntegerOverflow=off  RndMeth=Floor
  Cast3 : DataTypeConversion  OutDataTypeStr=int16  SaturateOnIntegerOverflow=off  RndMeth=Floor
  Mux : Mux
  Serial Transmit : arduinolib/Serial Transmit  portNumber=2  sendmode=write  sendformat=Decimal  floatprecision=2  header=[]  terminator=[]  blockPlatform=arduino
  Start Frame : Constant  Value=0xABCD  OutDataTypeStr=uint16
  wires:
  Cast1/1 -> Bitwise XOR1/3, Mux/3
  Speed Front/1 -> Cast3/1
  Start Frame/1 -> Bitwise XOR1/1, Mux/1
  Mux/1 -> Serial Transmit/1
  Steer Front/1 -> Cast2/1
  Bitwise XOR1/1 -> Mux/4
  Cast/1 -> Bitwise XOR1/2, Mux/2
  Cast2/1 -> Cast/1
  Cast3/1 -> Cast1/1

== system diff_controller/commands_rear_wheels ==
  Speed Rear : Inport
  Steer Rear : Inport  Port=2
  Bitwise XOR1 : simulink/Logic and Bit Operations/Bitwise Operator  logicop=XOR  UseBitMask=off  NumInputPorts=3  BitMask=bin2dec('11011001')  BitMaskRealWorld=Stored Integer
      settings: LibrarySourceBlock=|
      | simulink/Quick Insert/Logic and Bit
      | Operations/Bitwise XOR
  Cast : DataTypeConversion  OutDataTypeStr=uint16  SaturateOnIntegerOverflow=off  RndMeth=Floor
  Cast1 : DataTypeConversion  OutDataTypeStr=uint16  SaturateOnIntegerOverflow=off  RndMeth=Floor
  Cast2 : DataTypeConversion  OutDataTypeStr=int16  SaturateOnIntegerOverflow=off  RndMeth=Floor
  Cast3 : DataTypeConversion  OutDataTypeStr=int16  SaturateOnIntegerOverflow=off  RndMeth=Floor
  Mux : Mux
  Serial Transmit : arduinolib/Serial Transmit  portNumber=1  sendmode=write  sendformat=Decimal  floatprecision=2  header=[]  terminator=[]  blockPlatform=arduino
  Start Frame : Constant  Value=0xABCD  OutDataTypeStr=uint16
  wires:
  Cast1/1 -> Bitwise XOR1/3, Mux/3
  Speed Rear/1 -> Cast3/1
  Start Frame/1 -> Bitwise XOR1/1, Mux/1
  Mux/1 -> Serial Transmit/1
  Steer Rear/1 -> Cast2/1
  Bitwise XOR1/1 -> Mux/4
  Cast/1 -> Bitwise XOR1/2, Mux/2
  Cast2/1 -> Cast/1
  Cast3/1 -> Cast1/1

== system diff_controller/Encoders/Subsystem1 ==
  In1 : Inport
  Enable : EnablePort
  Data Store Write : DataStoreWrite  IndexOptions=Index vector (dialog)  Indices=1  OutputSizes=1
  wires:
  In1/1 -> Data Store Write/1

== system diff_controller/Encoders Left/Subsystem1 ==
  In1 : Inport
  Enable : EnablePort
  Data Store Write : DataStoreWrite  IndexOptions=Index vector (dialog)  Indices=1  OutputSizes=1
  wires:
  In1/1 -> Data Store Write/1

== system diff_controller/Encoders Left1/Subsystem1 ==
  In1 : Inport
  Enable : EnablePort
  Data Store Write : DataStoreWrite  IndexOptions=Index vector (dialog)  Indices=1  OutputSizes=1
  wires:
  In1/1 -> Data Store Write/1

== system diff_controller/Encoders Right/Subsystem1 ==
  In1 : Inport
  Enable : EnablePort
  Data Store Write : DataStoreWrite  IndexOptions=Index vector (dialog)  Indices=1  OutputSizes=1
  wires:
  In1/1 -> Data Store Write/1

== system diff_controller/Encoders Right1/Subsystem1 ==
  In1 : Inport
  Enable : EnablePort
  Data Store Write : DataStoreWrite  IndexOptions=Index vector (dialog)  Indices=1  OutputSizes=1
  wires:
  In1/1 -> Data Store Write/1

== system diff_controller/Encoders1/Subsystem1 ==
  In1 : Inport
  Enable : EnablePort
  Data Store Write : DataStoreWrite  IndexOptions=Index vector (dialog)  Indices=1  OutputSizes=1
  wires:
  In1/1 -> Data Store Write/1

== system diff_controller/Ref Parser/Subsystem1 ==
  In1 : Inport
  Enable : EnablePort
  Data Store Write : DataStoreWrite  IndexOptions=Index vector (dialog)  Indices=1  OutputSizes=1
  wires:
  In1/1 -> Data Store Write/1

== system diff_controller/Subsystem1/Subsystem1 ==
  In1 : Inport
  Enable : EnablePort
  Data Store Write : DataStoreWrite  IndexOptions=Index vector (dialog)  Indices=1  OutputSizes=1
  wires:
  In1/1 -> Data Store Write/1

== matlab function diff_controller/Encoders Left/Encoder Parser ==
  settings: updateMethod=DISCRETE  sampleTime=Ts
  data: data input; averageSpeed output
function averageSpeed = process_feedback(data)

% Feedback is sent every 10ms:
% 
% Start frame(unsigned int16) : 0xABCD
% Cmd1(signed int16) : Steer or Brake(hovercar) after normalizing and mixing
% Cmd2(signed int16) : Speed or Throttle(hovercar) after normalizing and mixing
% SpeedR(signed int16) : Measured right wheel speed in RPM
% SpeedL(signed int16) : Measured left wheel speed in RPM
% Battery Voltage(signed int16) : Calibrated Battery Voltage *100
% Temperature(signed int16) : Temperature in °C *10
% Led(unsigned int16) : Used to control the leds on the sideboard
% Checksum(unsigned int16) : XOR checksum
%
%

    persistent lastValidAverageSpeed;

    if isempty(lastValidAverageSpeed)
        lastValidAverageSpeed = int16(0); 
    end
    

    START_FRAME = int16(-21555);
    PACKET_SIZE = 9; 

    data = data(:)';

    for i = 1:(length(data) - PACKET_SIZE + 1)

        if data(i) == START_FRAME
            packet = data(i:(i + PACKET_SIZE - 1));

            Cmd1 = packet(2);
            Cmd2 = packet(3);
            Speed1 = packet(4);
            Speed2 = packet(5);
            BatteryVoltage = packet(6);
            Temperature = packet(7);

            %Note that the original data protocal, the Led is uint16.
            %To solve the data mismatch in the bitxor, we used int16.
            %Original: Led = uint16(packet(8));
            Led = packet(8);
            receivedChecksum = uint16(packet(9));
            
            computedChecksum = bitxor(START_FRAME, Cmd1);
            computedChecksum = bitxor(computedChecksum, Cmd2);
            computedChecksum = bitxor(computedChecksum, Speed1);
            computedChecksum = bitxor(computedChecksum, Speed2);
            computedChecksum = bitxor(computedChecksum, BatteryVoltage);
            computedChecksum = bitxor(computedChecksum, Temperature);
            
            %Data types mismatch. 
            computedChecksum = bitxor(computedChecksum, Led);

            if computedChecksum == receivedChecksum
                lastValidAverageSpeed = int16(mean([(abs(Speed1)), (abs(Speed2))]));
            end
        end
    end

    averageSpeed = lastValidAverageSpeed;
end

== stateflow chart diff_controller/Chart3 ==
  settings: updateMethod=DISCRETE  sampleTime=Ts
  state Moving
    entry:
    steer_right = (0.5*(base_speed+(desired_theta*width)/taw));
    speed_right = 0;
    steer_left = -(0.5*(base_speed-(desired_theta*width)/taw));
    speed_left = 0;
    during:
    steer_right = 0.5*(base_speed+(desired_theta*width)/taw);
    steer_left = -0.5*(base_speed-(desired_theta*width)/taw);
  state Init
    entry:
    steer_right = 0;
    speed_right = 0;
    steer_left = 0;
    speed_left = 0;
  state Stopped
    entry:
    steer_right = 0;
    speed_right = 0;
    steer_left = 0;
    speed_left = 0;
  (default) -> Init
  Init -> Moving : after(10,sec)
  Stopped -> Moving : [desired_distance > 1 || desired_distance < -1]
  Moving -> Stopped : [desired_distance <= 1 && desired_distance >= -1]
  data: speed_right output; desired_theta input; desired_distance input; steer_right output; speed_left output; steer_left output; taw input; base_speed input; width local =0.441

== stateflow chart diff_controller/Chart4 ==
  settings: updateMethod=DISCRETE  sampleTime=Ts
  state Moving
    entry:
    steer_right = 0;
    steer_left = 0;
    speed_right = 0.5*(base_speed+(desired_theta*width)/taw);
    speed_left = 0.5*(base_speed-(desired_theta*width)/taw);
    during:
    speed_right = 0.5*(base_speed+(desired_theta*width)/taw);
    speed_left = 0.5*(base_speed-(desired_theta*width)/taw);
  state Init
    entry:
    steer_right = 0;
    speed_right = 0;
    steer_left = 0;
    speed_left = 0;
  state Stopped
    entry:
    steer_right = 0;
    speed_right = 0;
    steer_left = 0;
    speed_left = 0;
  (default) -> Init
  Init -> Moving : after(10,sec)
  Stopped -> Moving : [desired_distance > 0.5 || desired_distance < -0.5]
  Moving -> Stopped : [desired_distance <= 0.5 && desired_distance >= -0.5]
  data: speed_right output; desired_theta input; desired_distance input; steer_right output; speed_left output; steer_left output; taw input; base_speed input; width local =0.441

== matlab function diff_controller/Encoders Left1/Encoder Parser ==
  settings: updateMethod=DISCRETE  sampleTime=Ts
  data: data input; averageSpeed output
function averageSpeed = process_feedback(data)

% Feedback is sent every 10ms:
% 
% Start frame(unsigned int16) : 0xABCD
% Cmd1(signed int16) : Steer or Brake(hovercar) after normalizing and mixing
% Cmd2(signed int16) : Speed or Throttle(hovercar) after normalizing and mixing
% SpeedR(signed int16) : Measured right wheel speed in RPM
% SpeedL(signed int16) : Measured left wheel speed in RPM
% Battery Voltage(signed int16) : Calibrated Battery Voltage *100
% Temperature(signed int16) : Temperature in °C *10
% Led(unsigned int16) : Used to control the leds on the sideboard
% Checksum(unsigned int16) : XOR checksum
%
%

    persistent lastValidAverageSpeed;

    if isempty(lastValidAverageSpeed)
        lastValidAverageSpeed = 0; 
    end
    

    START_FRAME = int16(-21555);
    PACKET_SIZE = 9; 

    data = data(:)';

    for i = 1:(length(data) - PACKET_SIZE + 1)

        if data(i) == START_FRAME
            packet = data(i:(i + PACKET_SIZE - 1));

            Cmd1 = packet(2);
            Cmd2 = packet(3);
            Speed1 = packet(4);
            Speed2 = packet(5);
            BatteryVoltage = packet(6);
            Temperature = packet(7);

            %Note that the original data protocal, the Led is uint16.
            %To solve the data mismatch in the bitxor, we used int16.
            %Original: Led = uint16(packet(8));
            Led = packet(8);
            receivedChecksum = uint16(packet(9));
            
            computedChecksum = bitxor(START_FRAME, Cmd1);
            computedChecksum = bitxor(computedChecksum, Cmd2);
            computedChecksum = bitxor(computedChecksum, Speed1);
            computedChecksum = bitxor(computedChecksum, Speed2);
            computedChecksum = bitxor(computedChecksum, BatteryVoltage);
            computedChecksum = bitxor(computedChecksum, Temperature);
            
            %Data types mismatch. 
            computedChecksum = bitxor(computedChecksum, Led);

            if computedChecksum == receivedChecksum
                lastValidAverageSpeed = mean([double(Speed1), double(Speed2)]);
            end
        end
    end

    averageSpeed = lastValidAverageSpeed;
end

== matlab function diff_controller/Encoders Right1/Encoder Parser ==
  settings: updateMethod=DISCRETE  sampleTime=Ts
  data: data input; averageSpeed output
function averageSpeed = process_feedback(data)

% Feedback is sent every 10ms:
% 
% Start frame(unsigned int16) : 0xABCD
% Cmd1(signed int16) : Steer or Brake(hovercar) after normalizing and mixing
% Cmd2(signed int16) : Speed or Throttle(hovercar) after normalizing and mixing
% SpeedR(signed int16) : Measured right wheel speed in RPM
% SpeedL(signed int16) : Measured left wheel speed in RPM
% Battery Voltage(signed int16) : Calibrated Battery Voltage *100
% Temperature(signed int16) : Temperature in °C *10
% Led(unsigned int16) : Used to control the leds on the sideboard
% Checksum(unsigned int16) : XOR checksum
%
%

    persistent lastValidAverageSpeed;

    if isempty(lastValidAverageSpeed)
        lastValidAverageSpeed = 0; 
    end
    

    START_FRAME = int16(-21555);
    PACKET_SIZE = 9; 

    data = data(:)';

    for i = 1:(length(data) - PACKET_SIZE + 1)

        if data(i) == START_FRAME
            packet = data(i:(i + PACKET_SIZE - 1));

            Cmd1 = packet(2);
            Cmd2 = packet(3);
            Speed1 = packet(4);
            Speed2 = packet(5);
            BatteryVoltage = packet(6);
            Temperature = packet(7);

            %Note that the original data protocal, the Led is uint16.
            %To solve the data mismatch in the bitxor, we used int16.
            %Original: Led = uint16(packet(8));
            Led = packet(8);
            receivedChecksum = uint16(packet(9));
            
            computedChecksum = bitxor(START_FRAME, Cmd1);
            computedChecksum = bitxor(computedChecksum, Cmd2);
            computedChecksum = bitxor(computedChecksum, Speed1);
            computedChecksum = bitxor(computedChecksum, Speed2);
            computedChecksum = bitxor(computedChecksum, BatteryVoltage);
            computedChecksum = bitxor(computedChecksum, Temperature);
            
            %Data types mismatch. 
            computedChecksum = bitxor(computedChecksum, Led);

            if computedChecksum == receivedChecksum
                lastValidAverageSpeed = mean([double(Speed1), double(Speed2)]);
            end
        end
    end

    averageSpeed = lastValidAverageSpeed;
end
